simulink model "autopilotstef_cessna172"  (R2015a)
settings: Solver=ode45  StartTime=0.0  StopTime=1000.0  RelTol=1e-3
libraries: FSD_Custom_BASE x1, X_Plane_Communication_Library x1, etargetslib x1, dspnetwork x1
settings Model: Creator=Stefan  LastModifiedBy=Stefan

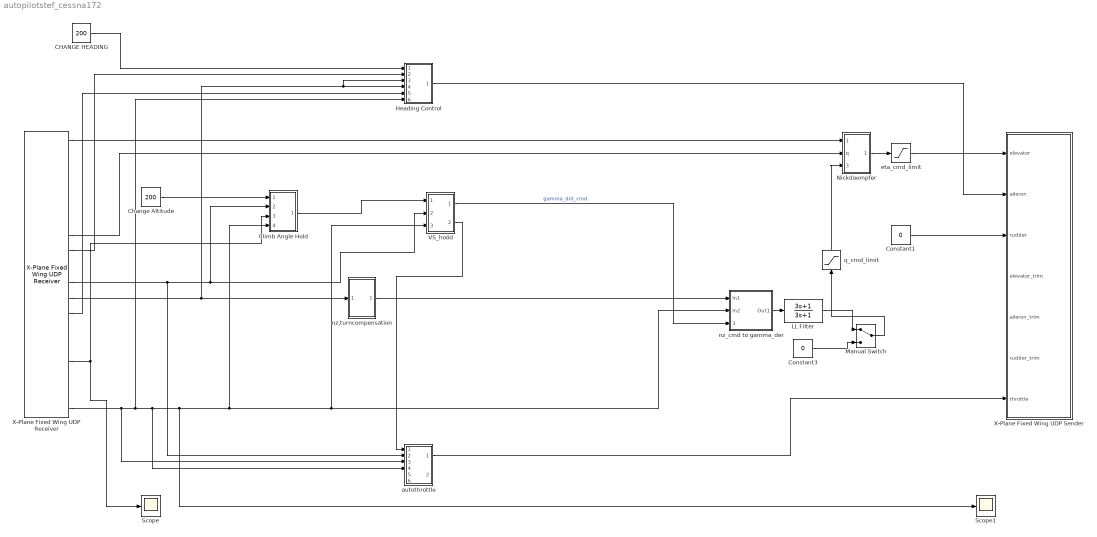
== system autopilotstef_cessna172 ==
  CHANGE HEADING : Constant  Value=200
  Change Altitude : Constant  Value=200
  Climb Angle Hold : Subsystem
  Constant1 : Constant  Value=0
  Constant3 : Constant  Value=0
  Heading Control : Subsystem
  LL Filter : TransferFcn  Numerator=[3 1]  Denominator=[3 1]
  Manual Switch : ManualSwitch
  Nickdaempfer : Subsystem
  Scope : Scope
      settings: YMin=0  YMax=4500  SaveName=ScopeData2
  Scope1 : Scope
      settings: YMin=90  YMax=130  SaveName=ScopeData3
  VS_hoöd : Subsystem
  X-Plane Fixed Wing UDP Receiver : X_Plane_Communication_Library/Fixed Wing/X-Plane Fixed Wing UDP Receiver  ip_adress='127.0.0.1'  port_number=49004
  X-Plane Fixed Wing UDP Sender : Subsystem  RequirementInfo="{}  %GIDa_a408a53f_2494_4354_a334_ac5c54aa80f1"  AncestorBlock=X_Plane_Communication_Library/Fixed Wing/X-Plane Fixed Wing UDP Sender  mask{ip_adress='127.0.0.1', port_number=49000}
      mask prompts: ip_adress "Local IP Adress (default: '127.0.0.1' )"; port_number "Output Port Number (defaut: '49000')"
      mask help: This block is configured to send data to a fixed wing aircraft on X-Plane Flight Simulator.
      mask Help: Contact adrianobittar@gmail.com
  autothrottle : Subsystem
  eta_cmd_limit : Saturate  UpperLimit=0.2  LowerLimit=-0.2
  nz,turncompensation : Subsystem
  nz_cmd to gamma_der : Subsystem
  q_cmd_limit : Saturate  UpperLimit=15*pi/180  LowerLimit=-15*pi/180
  wires:
  Constant1/1 -> X-Plane Fixed Wing UDP Sender/3(rudder)
  X-Plane Fixed Wing UDP Receiver/1 -> Nickdaempfer/1(elevator)
  X-Plane Fixed Wing UDP Receiver/7 -> Nickdaempfer/2(q)
  Nickdaempfer/1("etta_cmd ") -> eta_cmd_limit/1
  X-Plane Fixed Wing UDP Receiver/11 -> Heading Control/4(In4), Heading Control/3(In3), nz,turncompensation/1(In1)
  nz,turncompensation/1(Out1) -> nz_cmd to gamma_der/1(In1)
  nz_cmd to gamma_der/1(Out1) -> LL Filter/1
  X-Plane Fixed Wing UDP Receiver/10 -> autothrottle/2(In2), Climb Angle Hold/2(In2), VS_hoöd/2(In2)
  VS_hoöd/1(Out1) -> nz_cmd to gamma_der/3("gamma_cmd ")  "gamma_dot_cmd"
  VS_hoöd/2(Out2) -> autothrottle/1(In1)
  autothrottle/1(Out1) -> X-Plane Fixed Wing UDP Sender/7(throttle)
  X-Plane Fixed Wing UDP Receiver/15 -> Climb Angle Hold/3(In3), Scope/1
  q_cmd_limit/1 -> Nickdaempfer/3(q_cmd)
  LL Filter/1 -> Manual Switch/1
  Manual Switch/1 -> q_cmd_limit/1
  Constant3/1 -> Manual Switch/2
  X-Plane Fixed Wing UDP Receiver/18 -> autothrottle/3(In3), Heading Control/6(In6), autothrottle/4(In4), Scope1/1, Climb Angle Hold/4(In4), nz_cmd to gamma_der/2(In2), VS_hoöd/3(In3)
  CHANGE HEADING/1 -> Heading Control/1(In1)
  X-Plane Fixed Wing UDP Receiver/8 -> Heading Control/2(In2)
  X-Plane Fixed Wing UDP Receiver/12 -> Heading Control/5(In5)
  Heading Control/1(Out1) -> X-Plane Fixed Wing UDP Sender/2(aileron)
  eta_cmd_limit/1 -> X-Plane Fixed Wing UDP Sender/1(elevator)
  Change Altitude/1 -> Climb Angle Hold/1(In1)
  Climb Angle Hold/1(Out1) -> VS_hoöd/1(In1)

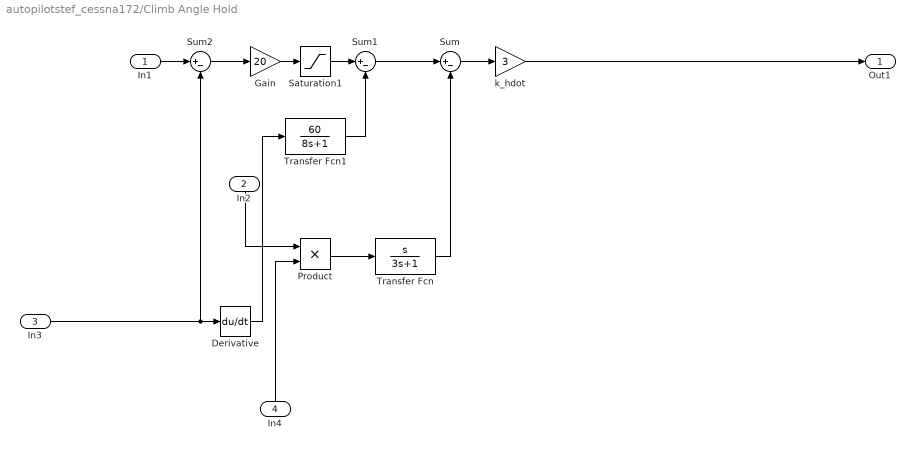
== system autopilotstef_cessna172/Climb Angle Hold ==
  In1 : Inport
  In2 : Inport  Port=2
  In3 : Inport  Port=3
  In4 : Inport  Port=4
  Derivative : Derivative
  Gain : Gain  Gain=20
  Product : Product
  Saturation1 : Saturate  UpperLimit=300  LowerLimit=-300
  Sum : Sum  Inputs=|+-
  Sum1 : Sum  Inputs=|+-
  Sum2 : Sum  Inputs=|+-
  Transfer Fcn : TransferFcn  Numerator=[1 0]  Denominator=[3 1]
  Transfer Fcn1 : TransferFcn  Numerator=[60]  Denominator=[8 1]
  k_hdot : Gain  Gain=3
  Out1 : Outport
  wires:
  In1/1 -> Sum2/1
  Saturation1/1 -> Sum1/1
  Sum2/1 -> Gain/1
  Sum/1 -> k_hdot/1
  Transfer Fcn1/1 -> Sum1/2
  Gain/1 -> Saturation1/1
  Transfer Fcn/1 -> Sum/2
  k_hdot/1 -> Out1/1
  Sum1/1 -> Sum/1
  Derivative/1 -> Transfer Fcn1/1
  Product/1 -> Transfer Fcn/1
  In3/1 -> Sum2/2, Derivative/1
  In2/1 -> Product/1
  In4/1 -> Product/2

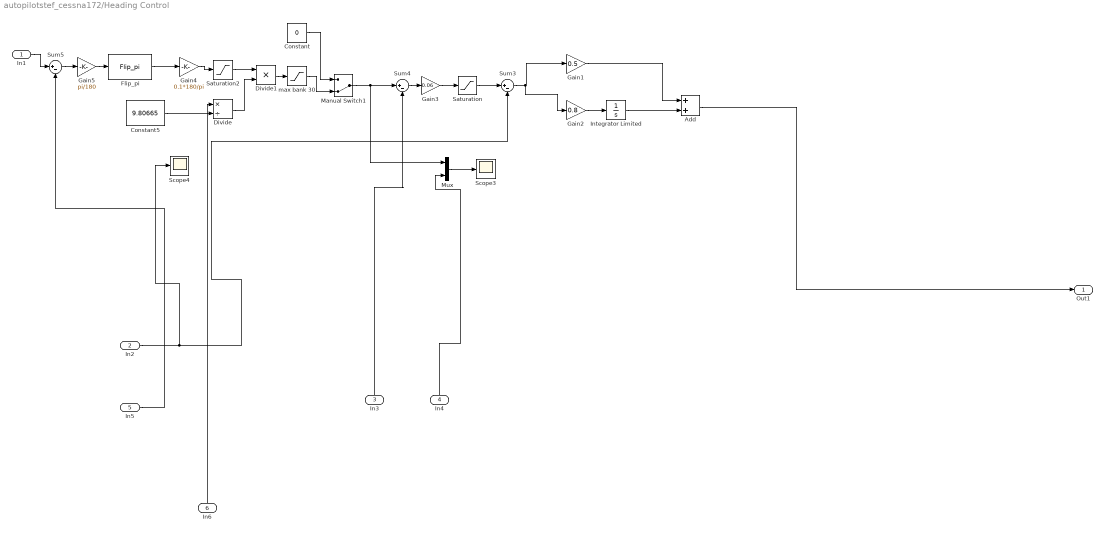
== system autopilotstef_cessna172/Heading Control ==
  In1 : Inport
  In2 : Inport  Port=2
  In3 : Inport  Port=3
  In4 : Inport  Port=4
  In5 : Inport  Port=5
  In6 : Inport  Port=6
  Add : Sum
  Constant : Constant  Value=0
  Constant5 : Constant  Value=9.80665
  Divide : Product  Inputs=*/
  Divide1 : Product  Inputs=**
  Flip_pi : FSD_Custom_BASE/Flip_pi
  Gain1 : Gain  Gain=0.5
  Gain2 : Gain  Gain=0.8
  Gain3 : Gain  Gain=0.06
  Gain4 : Gain  Gain=0.1*180/pi
  Gain5 : Gain  Gain=pi/180
  Integrator Limited : Integrator  LimitOutput=on  UpperSaturationLimit=0.7  LowerSaturationLimit=-0.7
  Manual Switch1 : ManualSwitch  CurrentSetting=0
  Mux : Mux  Inputs=2
  Saturation : Saturate  UpperLimit=4  LowerLimit=-4
  Saturation2 : Saturate  UpperLimit=3  LowerLimit=-3
  Scope3 : Scope
      settings: YMin=0  YMax=50  SaveName=ScopeData5
  Scope4 : Scope
      settings: YMin=-0.01  YMax=0.07  SaveName=ScopeData6
  Sum3 : Sum  Inputs=|+-
  Sum4 : Sum  Inputs=|+-
  Sum5 : Sum  Inputs=|+-
  max bank 30 : Saturate  UpperLimit=30  LowerLimit=-30
  Out1 : Outport
  wires:
  Divide1/1 -> max bank 30/1
  Mux/1 -> Scope3/1
  Divide/1 -> Divide1/2
  In3/1 -> Sum4/2
  In6/1 -> Divide/1
  In4/1 -> Mux/2
  Gain4/1 -> Saturation2/1
  Flip_pi/1 -> Gain4/1
  Saturation2/1 -> Divide1/1
  In1/1 -> Sum5/1
  Constant5/1 -> Divide/2
  Gain5/1 -> Flip_pi/1
  Sum5/1 -> Gain5/1
  In5/1 -> Sum5/2
  Gain3/1 -> Saturation/1
  Saturation/1 -> Sum3/1
  Sum3/1 -> Gain2/1, Gain1/1
  Gain1/1 -> Add/1
  Add/1 -> Out1/1
  Constant/1 -> Manual Switch1/1
  In2/1 -> Scope4/1, Sum3/2
  max bank 30/1 -> Manual Switch1/2
  Integrator Limited/1 -> Add/2
  Manual Switch1/1 -> Mux/1, Sum4/1
  Gain2/1 -> Integrator Limited/1
  Sum4/1 -> Gain3/1

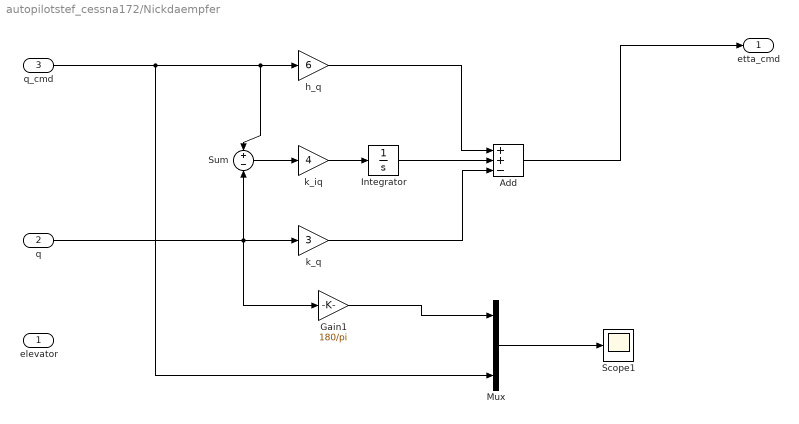
== system autopilotstef_cessna172/Nickdaempfer ==
  elevator : Inport
  q : Inport  Port=2
  q_cmd : Inport  Port=3
  Add : Sum  Inputs=++-
  Gain1 : Gain  Gain=180/pi
  Integrator : Integrator
  Mux : Mux
  Scope1 : Scope
      settings: TimeRange=100  YMin=-4.5  YMax=3.5
  Sum : Sum  Inputs=+|-
  h_q : Gain  Gain=6
  k_iq : Gain  Gain=4
  k_q : Gain  Gain=3
  "etta_cmd " : Outport
  wires:
  Mux/1 -> Scope1/1
  k_q/1 -> Add/3
  k_iq/1 -> Integrator/1
  Sum/1 -> k_iq/1
  h_q/1 -> Add/1
  Integrator/1 -> Add/2
  Add/1 -> "etta_cmd "/1
  q/1 -> Gain1/1, Sum/2, k_q/1
  Gain1/1 -> Mux/1
  q_cmd/1 -> Sum/1, h_q/1, Mux/4

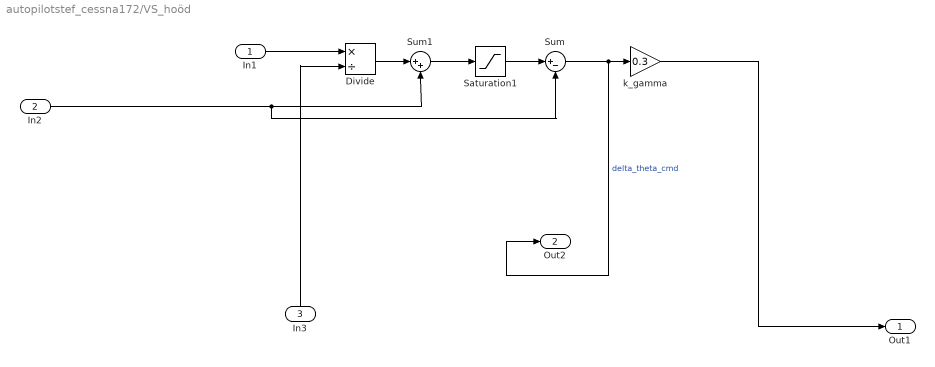
== system autopilotstef_cessna172/VS_hoöd ==
  In1 : Inport
  In2 : Inport  Port=2
  In3 : Inport  Port=3
  Divide : Product  Inputs=*/
  Saturation1 : Saturate  UpperLimit=6  LowerLimit=-15
  Sum : Sum  Inputs=|+-
  Sum1 : Sum  Inputs=|++
  k_gamma : Gain  Gain=0.3
  Out1 : Outport
  Out2 : Outport  Port=2
  wires:
  Sum1/1 -> Saturation1/1
  k_gamma/1 -> Out1/1
  In3/1 -> Divide/2
  In2/1 -> Sum1/2, Sum/2
  In1/1 -> Divide/1
  Divide/1 -> Sum1/1
  Sum/1 -> Out2/1, k_gamma/1  "delta_theta_cmd"
  Saturation1/1 -> Sum/1

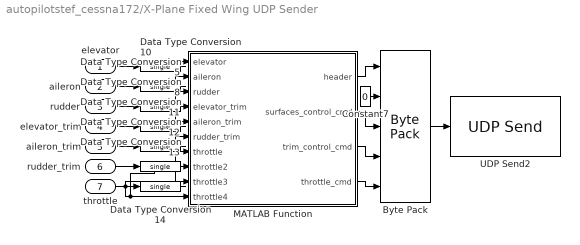
== system autopilotstef_cessna172/X-Plane Fixed Wing UDP Sender ==
  elevator : Inport
  aileron : Inport  Port=2
  rudder : Inport  Port=3
  elevator_trim : Inport  Port=4
  aileron_trim : Inport  Port=5
  rudder_trim : Inport  Port=6
  throttle : Inport  Port=7
  Byte Pack : etargetslib/Byte Pack  datatypes={'single','uint8','single','single','single'}  byteAlign=1
  Constant7 : Constant  Value=0  OutDataTypeStr=uint8
  Data Type Conversion{5,8,10..14} (7 alike) : DataTypeConversion  OutDataTypeStr=single  SaturateOnIntegerOverflow=on
  MATLAB Function : MATLAB Function  TreatAsAtomicUnit=on
  UDP Send2 : dspnetwork/UDP Send  remoteURL=ip_adress  remotePort=port_number  localURL='255.255.255.255'  localPortSource=Automatically determine  localPort=-1  sampletime=-1  blockPlatform=HOST  separateLengthPort=0
  wires:
  rudder_trim/1 -> Data Type Conversion13/1
  MATLAB Function/2(surfaces_control_cmd) -> Byte Pack/3
  Byte Pack/1 -> UDP Send2/1
  elevator_trim/1 -> Data Type Conversion11/1
  MATLAB Function/1(header) -> Byte Pack/1
  Data Type Conversion12/1 -> MATLAB Function/5(aileron_trim)
  Data Type Conversion13/1 -> MATLAB Function/6(rudder_trim)
  aileron_trim/1 -> Data Type Conversion12/1
  MATLAB Function/3(trim_control_cmd) -> Byte Pack/4
  Data Type Conversion14/1 -> MATLAB Function/7(throttle)
  Data Type Conversion5/1 -> MATLAB Function/2(aileron)
  MATLAB Function/4(throttle_cmd) -> Byte Pack/5
  elevator/1 -> Data Type Conversion10/1
  aileron/1 -> Data Type Conversion5/1
  Data Type Conversion11/1 -> MATLAB Function/4(elevator_trim)
  Data Type Conversion10/1 -> MATLAB Function/1(elevator)
  throttle/1 -> MATLAB Function/9(throttle3), Data Type Conversion14/1, MATLAB Function/8(throttle2), MATLAB Function/10(throttle4)
  Data Type Conversion8/1 -> MATLAB Function/3(rudder)
  Constant7/1 -> Byte Pack/2
  rudder/1 -> Data Type Conversion8/1

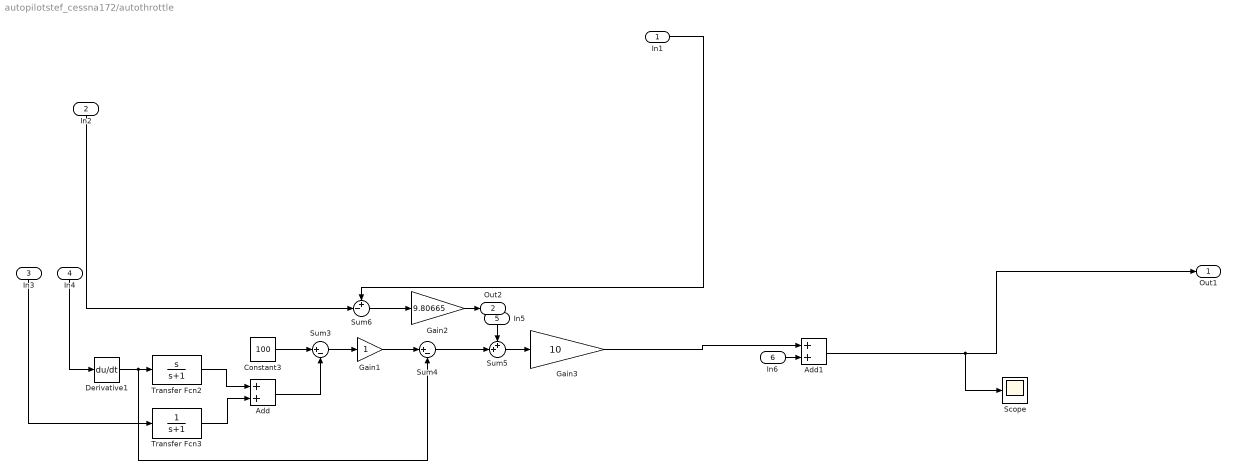
== system autopilotstef_cessna172/autothrottle ==
  In1 : Inport
  In2 : Inport  Port=2
  In3 : Inport  Port=3
  In4 : Inport  Port=4
  In5 : Inport  Port=5
  In6 : Inport  Port=6
  Add : Sum
  Add1 : Sum
  Constant3 : Constant  Value=100
  Derivative1 : Derivative
  Gain1 : Gain
  Gain2 : Gain  Gain=9.80665
  Gain3 : Gain  Gain=10
  Scope : Scope
      settings: YMin=-10  YMax=32.5
  Sum3 : Sum  Inputs=|+-
  Sum4 : Sum  Inputs=|+-
  Sum5 : Sum  Inputs=++|
  Sum6 : Sum  Inputs=+-|
  Transfer Fcn2 : TransferFcn  Numerator=[1 0]  Denominator=[1 1]
  Transfer Fcn3 : TransferFcn  Denominator=[1 1]
  Out1 : Outport
  Out2 : Outport  Port=2
  wires:
  Add/1 -> Sum3/2
  Transfer Fcn2/1 -> Add/1
  Sum5/1 -> Gain3/1
  In1/1 -> Sum6/1
  Gain3/1 -> Add1/1
  Transfer Fcn3/1 -> Add/2
  Sum6/1 -> Gain2/1
  Gain1/1 -> Sum4/1
  Sum4/1 -> Sum5/2
  Constant3/1 -> Sum3/1
  Sum3/1 -> Gain1/1
  Derivative1/1 -> Sum4/2, Transfer Fcn2/1
  In5/1 -> Sum5/1
  In4/1 -> Derivative1/1
  In2/1 -> Sum6/2
  In6/1 -> Add1/2
  Gain2/1 -> Out2/1
  In3/1 -> Transfer Fcn3/1
  Add1/1 -> Out1/1, Scope/1

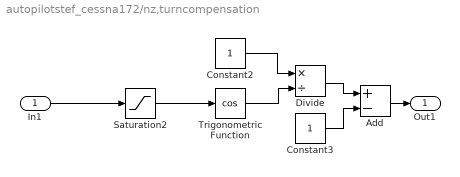
== system autopilotstef_cessna172/nz,turncompensation ==
  In1 : Inport
  Add : Sum  Inputs=+-
  Constant2 : Constant
  Constant3 : Constant
  Divide : Product  Inputs=*/
  Saturation2 : Saturate  UpperLimit=30*pi/180  LowerLimit=-30*pi/180
  Trigonometric Function : Trigonometry  Operator=cos
  Out1 : Outport
  wires:
  Trigonometric Function/1 -> Divide/2
  In1/1 -> Saturation2/1
  Constant2/1 -> Divide/1
  Constant3/1 -> Add/2
  Saturation2/1 -> Trigonometric Function/1
  Add/1 -> Out1/1
  Divide/1 -> Add/1

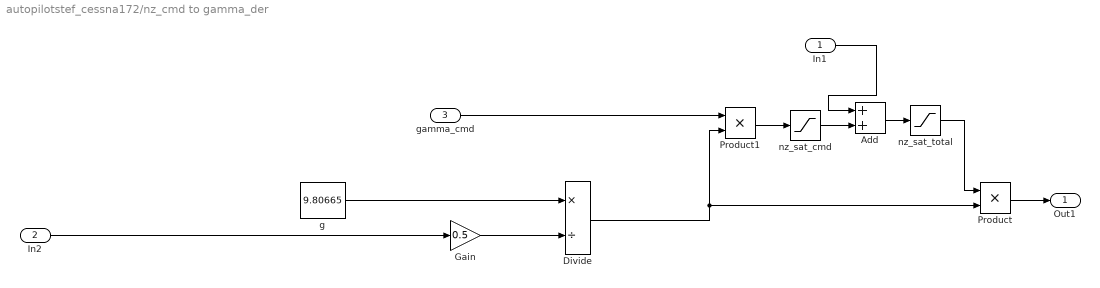
== system autopilotstef_cessna172/nz_cmd to gamma_der ==
  In1 : Inport
  In2 : Inport  Port=2
  "gamma_cmd " : Inport  Port=3
  Add : Sum
  Divide : Product  Inputs=*/
  Gain : Gain  Gain=0.5
  Product : Product
  Product1 : Product
  "g " : Constant  Value=9.80665
  nz_sat_cmd : Saturate  UpperLimit=2  LowerLimit=-2
  nz_sat_total : Saturate  UpperLimit=4  LowerLimit=-4
  Out1 : Outport
  wires:
  Product/1 -> Out1/1
  "gamma_cmd "/1 -> Product1/1
  nz_sat_total/1 -> Product/1
  Divide/1 -> Product/2, Product1/2
  In2/1 -> Gain/1
  nz_sat_cmd/1 -> Add/2
  Product1/1 -> nz_sat_cmd/1
  In1/1 -> Add/1
  Add/1 -> nz_sat_total/1
  "g "/1 -> Divide/1
  Gain/1 -> Divide/2

== matlab function autopilotstef_cessna172/X-Plane Fixed Wing UDP Sender/MATLAB Function ==
  data: elevator input single size=1; aileron input; rudder input; elevator_trim input; aileron_trim input; rudder_trim input; throttle input; header output single size=1; surfaces_control_cmd output single size=[1 18]; trim_control_cmd output single size=[1 18]; throttle_cmd output size=[1 18]; throttle2 input; throttle3 input; throttle4 input
function [header, surfaces_control_cmd,trim_control_cmd, throttle_cmd]  = fcn(elevator, aileron, rudder, elevator_trim, aileron_trim, rudder_trim, throttle, throttle2, throttle3, throttle4)
% This block supports the Embedded MATLAB subset.
% See the help menu for details. 

header = typecast(uint8([uint8(68) uint8(65) uint8(84) uint8(65)]), 'single');



No_Comand = single(-999);

Surface_header = typecast(uint8([uint8(8) uint8(0) uint8(0) uint8(0)]), 'single');

surfaces_control_cmd = [Surface_header elevator aileron rudder No_Comand No_Comand No_Comand No_Comand No_Comand Surface_header No_Comand No_Comand No_Comand No_Comand No_Comand No_Comand No_Comand No_Comand];

Trim_header = typecast(uint8([uint8(13) uint8(0) uint8(0) uint8(0)]), 'single');


trim_control_cmd = [ Trim_header elevator_trim aileron_trim rudder_trim No_Comand No_Comand No_Comand No_Comand No_Comand Trim_header No_Comand No_Comand No_Comand No_Comand No_Comand No_Comand No_Comand No_Comand];

Throttle_header = typecast(uint8([uint8(25) uint8(0) uint8(0) uint8(0)]), 'single');
throttle_cmd = [Throttle_header throttle throttle2 throttle3 throttle4 No_Comand No_Comand No_Comand No_Comand Throttle_header No_Comand No_Comand No_Comand No_Comand No_Comand No_Comand No_Comand No_Comand];




% Actuadors_Out[0] = 68;
% Actuadors_Out[1] = 65;
% Actuadors_Out[2] = 84;
% Actuadors_Out[3] = 65;
% Actuadors_Out[4] = 48;//26;
% aileron = data_in(3,1);
% rudder= data_in(4,1);
% 
% 
% elevator_trim= data_in(2,2);
% aileron_trim= data_in(3,2);
% rudder_trim= data_in(4,2);
% 
% q= data_in(2,3);
% p= data_in(3,3);
% r= data_in(4,3);
% 
% pitch= data_in(2,4);
% roll= data_in(3,4);
% heading_true= data_in(4,4);
% 
% Px= data_in(2,5);
% Py= data_in(3,5);
% Pz= data_in(4,5);
% Vx= data_in(5,5);
% Vy= data_in(6,5);
% Vz= data_in(7,5);
% 
% collective_main= data_in(2,6);
% collective_tail= data_in(3,6);
